simulink model "TV_2018_HIL"  (R2016a)
settings: Solver=FixedStepAuto  StartTime=0.0  StopTime=inf  FixedStep=0.001  RelTol=1e-3
PreLoadFcn:
  | TV_2017_parameters
values from neighbouring files (symbols this model uses):
  battery_voltage = single(530)    [HIL_parameters.m]    (also in HIL_parameters_2018.m; TV_2017_parameters.m; TV_2017_parameters_VD.m)
  car_params = Simulink_Car_params    [HIL_parameters.m]    (also in HIL_parameters_2018.m; TV_2017_parameters.m; TV_2017_parameters_VD.m)
  i_Diff = 16    [HIL_parameters.m]    (also in HIL_parameters_2018.m; TV_2017_parameters.m)
  Kp = 1    [HIL_parameters.m]    (also in HIL_parameters_2018.m; TV_2017_parameters.m; TV_2017_parameters_VD.m)
  motor_data = struct    [HIL_parameters.m]    (also in HIL_parameters_2018.m; TV_2017_parameters.m)
  powerLimitControl = Simulink_el    [HIL_parameters.m]    (also in HIL_parameters_2018.m; TV_2017_parameters.m; TV_2017_parameters_VD.m)
  settings = Simulink_Settings    [HIL_parameters.m]    (also in HIL_parameters_2018.m; TV_2017_parameters.m; TV_2017_parameters_VD.m)
  SpdC_BCC = 0    [HIL_parameters.m]    (also in HIL_parameters_2018.m; TV_2017_parameters.m; TV_2017_parameters_VD.m)
  Speed_Neg_sat = -21    [HIL_parameters.m]    (also in HIL_parameters_2018.m; TV_2017_parameters.m; TV_2017_parameters_VD.m)
  Speed_Pos_sat = 21    [HIL_parameters.m]    (also in HIL_parameters_2018.m; TV_2017_parameters.m; TV_2017_parameters_VD.m)
  SteeringAngleFL = [-23.80 -22.65 -21.50 -20.34 -19.18 -18.03 -16.86 -15.70 -14.53 -13.35 -12.18 -10.99 -9.80 -8.61 -7.40 -6.19 -4.97 -3.75 -2.51 -1.26 0 1.27 2.56 3.85 5.17 6.50 7.84 9.21 10.59 12.00 13.42 14.88 16.36 17.87 19.41 20.99 22.61 24.26 25.97 27.73 29.54]    [CarSetupAnalysis2018.m]    (also in HIL_parameters_2018.m; TV_2017_parameters.m; TV_2017_parameters_VD.m = [-24.129 -22.950 -21.772 -20.593 -19.413 -18.232 -17.050 -15)
  SteeringAngleFR = [-29.54 -27.73 -25.97 -24.26 -22.61 -20.99 -19.41 -17.87 -16.36 -14.88 -13.42 -12.00 -10.59 -9.21 -7.84 -6.50 -5.17 -3.85 -2.56 -1.27 0 1.26 2.51 3.75 4.97 6.19 7.40 8.61 9.80 10.99 12.18 13.35 14.53 15.70 16.86 18.03 19.18 20.34 21.50 22.65 23.80]    [CarSetupAnalysis2018.m]    (also in HIL_parameters_2018.m; TV_2017_parameters.m; TV_2017_parameters_VD.m = [-29.3050 -27.5340 -25.8140 -24.1410 -22.5110 -20.9180 -19.3)
  SteeringWhAngle = [-105 -99.75 -94.5 -89.25 -84 -78.75 -73.5 -68.25 -63 -57.75 -52.5 -47.25 -42 -36.75 -31.5 -26.25 -21.0 -15.75 -10.5 -5.25 0.0 5.25 10.50 15.75 21.00 26.25 31.50 36.75 42.00 47.25 52.50 57.75  63.00 68.25 73.50 78.75 84.00 89.25 94.50 99.75 105.00]    [TV_2017_parameters_VD.m]
  Tn_n = 0    [HIL_parameters.m]    (also in HIL_parameters_2018.m; TV_2017_parameters.m; TV_2017_parameters_VD.m)
  tractionControl = Simulink_tc    [HIL_parameters.m]    (also in HIL_parameters_2018.m; IterativeTractionControlTuning.m; TV_2017_parameters.m; TV_2017_parameters_VD.m)
  yawMomentGenerator = struct    [HIL_parameters.m]    (also in HIL_parameters_2018.m = Simulink_yawRate2; TV_2017_parameters.m = Simulink_yawRate2)
  yawRateControl = Simulink_yawRate    [HIL_parameters.m]    (also in HIL_parameters_2018.m; TV_2017_parameters.m; TV_2017_parameters_VD.m)
undefined symbols (not defined in the file or in its folder): canChannel, DiscIntNeverNeededParam, magnitude, speedEstimation, TC_Decr_Gas, TC_Derivative, TC_Incr_Gas, TC_On, TC_Relay_Off, TC_Relay_On
libraries: CarMaker4SL x366, simulink_extras x63, canmsglib x55, canlib x41, simulink x37, dspfdesign x2, sldrtlib x1
(part 2 of 15)

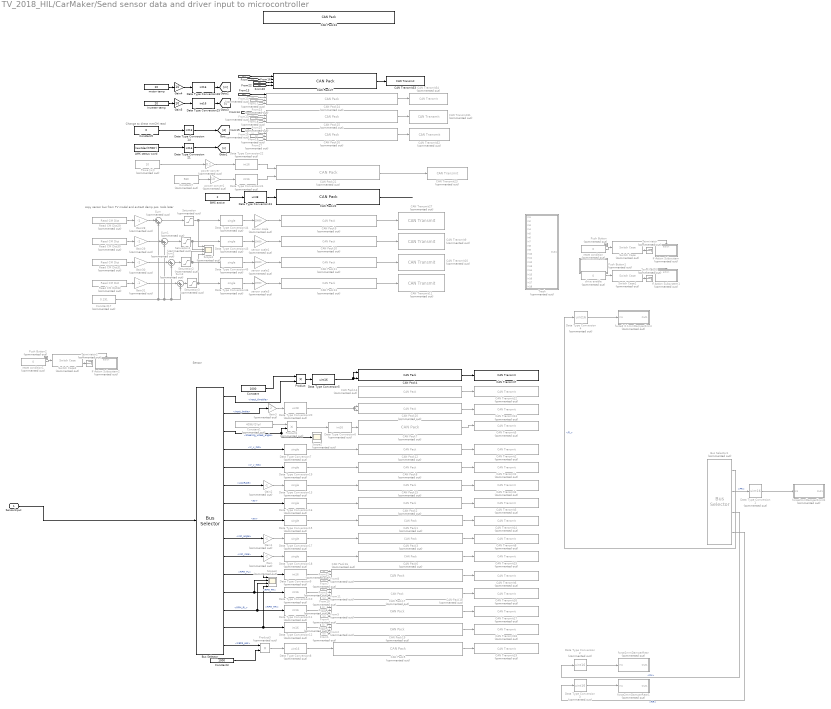
== system TV_2018_HIL/CarMaker/Send sensor data and driver input to microcontroller  ==
  note: Sensor
  note: copy sensor bus from TV model and extract damp pos. todo later
  note: Change to direct mmCM read
  SensorInput : Inport
  AMK status word : Constant  Value=hex2dec('F900')
  "BMS active " : Constant  Value=2
  Bus Selector : BusSelector  OutputSignals=Input_throttle,Input_brake,steering_wheel_angle,V_x_INS,V_y_INS,yawRate,ay,ax,roll_angle,roll_rate,RPM_FL,RPM_FR,RPM_RL,RPM_RR,KERS_pos
  Bus Selector1 : BusSelector  Commented=on  OutputSignals=FL,FR,RL,RR
  CAN Pack1 : canmsglib/CAN Pack  Commented=on  MsgList=(none)  MsgName=CAN Msg  MsgIDType=Standard (11-bit identifier)  MsgIdentifier=INS_A_X_ID  MsgLength=4  SignalInfo=Signal1$0$32$1$3$1$0$1$0$-Inf$Inf$#  NSignals=1  StartBits=str2num('[int32(0)]')  SignalSizes=str2num('[int32(32)]')  ByteOrders=str2num('[int32(1)]')  DataTypes=str2num('[int32(3)]')  MultiplexTypes=str2num('[int32(1)]')  MultiplexValues=str2num('[double(0)]')  Factors=str2num('[double(1)]')  Offsets=str2num('[double(0)]')  Minimums=str2num('[double(-Inf)]')  Maximums=str2num('[double(Inf)]')  Remote=off
      settings: DataFormat=manually specified signals
  CAN Pack10 : canmsglib/CAN Pack  Commented=on  MsgList=(none)  MsgName=ACD_DAMPER_FR_ID  MsgIDType=Standard (11-bit identifier)  MsgIdentifier=ACD_DAMPER_FR_ID  MsgLength=2  SignalInfo=Signal1$0$16$1$1$1$0$1$0$-Inf$Inf$#  NSignals=1  StartBits=str2num('[int32(0)]')  SignalSizes=str2num('[int32(16)]')  ByteOrders=str2num('[int32(1)]')  DataTypes=str2num('[int32(1)]')  MultiplexTypes=str2num('[int32(1)]')  MultiplexValues=str2num('[double(0)]')  Factors=str2num('[double(1)]')  Offsets=str2num('[double(0)]')  Minimums=str2num('[double(-Inf)]')  Maximums=str2num('[double(Inf)]')  Remote=off
      settings: DataFormat=manually specified signals
  CAN Pack11 : canmsglib/CAN Pack  Commented=on  MsgList=(none)  MsgName=ACD_DAMPER_RL_ID  MsgIDType=Standard (11-bit identifier)  MsgIdentifier=ACD_DAMPER_RL_ID  MsgLength=2  SignalInfo=Signal1$0$16$1$1$1$0$1$0$-Inf$Inf$#  NSignals=1  StartBits=str2num('[int32(0)]')  SignalSizes=str2num('[int32(16)]')  ByteOrders=str2num('[int32(1)]')  DataTypes=str2num('[int32(1)]')  MultiplexTypes=str2num('[int32(1)]')  MultiplexValues=str2num('[double(0)]')  Factors=str2num('[double(1)]')  Offsets=str2num('[double(0)]')  Minimums=str2num('[double(-Inf)]')  Maximums=str2num('[double(Inf)]')  Remote=off
      settings: DataFormat=manually specified signals
  CAN Pack12 : canmsglib/CAN Pack  Commented=on  MsgList=(none)  MsgName=CAN Msg  MsgIDType=Standard (11-bit identifier)  MsgIdentifier=INS_V_X_ID  MsgLength=4  SignalInfo=Signal1$0$32$1$3$1$0$1$0$-Inf$Inf$#  NSignals=1  StartBits=str2num('[int32(0)]')  SignalSizes=str2num('[int32(32)]')  ByteOrders=str2num('[int32(1)]')  DataTypes=str2num('[int32(3)]')  MultiplexTypes=str2num('[int32(1)]')  MultiplexValues=str2num('[double(0)]')  Factors=str2num('[double(1)]')  Offsets=str2num('[double(0)]')  Minimums=str2num('[double(-Inf)]')  Maximums=str2num('[double(Inf)]')  Remote=off
      settings: DataFormat=manually specified signals
  CAN Pack13 : canmsglib/CAN Pack  Commented=on  MsgList=(none)  MsgName=ACD_DAMPER_RR_ID  MsgIDType=Standard (11-bit identifier)  MsgIdentifier=ACD_DAMPER_RR_ID  MsgLength=2  SignalInfo=Signal1$0$16$1$1$1$0$1$0$-Inf$Inf$#  NSignals=1  StartBits=str2num('[int32(0)]')  SignalSizes=str2num('[int32(16)]')  ByteOrders=str2num('[int32(1)]')  DataTypes=str2num('[int32(1)]')  MultiplexTypes=str2num('[int32(1)]')  MultiplexValues=str2num('[double(0)]')  Factors=str2num('[double(1)]')  Offsets=str2num('[double(0)]')  Minimums=str2num('[double(-Inf)]')  Maximums=str2num('[double(Inf)]')  Remote=off
      settings: DataFormat=manually specified signals
  CAN Pack14 : canmsglib/CAN Pack  Commented=on  MsgList=(none)  MsgName=CAN Msg  MsgIDType=Standard (11-bit identifier)  MsgIdentifier=ADC_TORQUE_POSITION_RIGHT_ID  MsgLength=2  SignalInfo=APPS_R$0$16$1$2$1$0$1$0$-Inf$Inf$#  NSignals=1  StartBits=str2num('[int32(0)]')  SignalSizes=str2num('[int32(16)]')  ByteOrders=str2num('[int32(1)]')  DataTypes=str2num('[int32(2)]')  MultiplexTypes=str2num('[int32(1)]')  MultiplexValues=str2num('[double(0)]')  Factors=str2num('[double(1)]')  Offsets=str2num('[double(0)]')  Minimums=str2num('[double(-Inf)]')  Maximums=str2num('[double(Inf)]')  Remote=off
      settings: DataFormat=manually specified signals
  CAN Pack15 : canmsglib/CAN Pack  Commented=on  MsgList=(none)  MsgName=CAN Msg  MsgIDType=Standard (11-bit identifier)  MsgIdentifier=INS_YAW_RATE_ID  MsgLength=4  SignalInfo=Signal1$0$32$1$3$1$0$1$0$-Inf$Inf$#  NSignals=1  StartBits=str2num('[int32(0)]')  SignalSizes=str2num('[int32(32)]')  ByteOrders=str2num('[int32(1)]')  DataTypes=str2num('[int32(3)]')  MultiplexTypes=str2num('[int32(1)]')  MultiplexValues=str2num('[double(0)]')  Factors=str2num('[double(1)]')  Offsets=str2num('[double(0)]')  Minimums=str2num('[double(-Inf)]')  Maximums=str2num('[double(Inf)]')  Remote=off
      settings: DataFormat=manually specified signals
  CAN Pack16 : canmsglib/CAN Pack  Commented=on  MsgList=(none)  MsgName=AMK Actual Values 1  MsgIDType=Standard (11-bit identifier)  MsgIdentifier=AMK_DATA_ACTUAL_VALUE_1_FL_ID  MsgLength=8  SignalInfo=AMK_Status$0$16$1$1$1$0$1$0$-Inf$Inf$#AMK_ActualVelocity$16$16$1$1$1$0$1$0$-Inf$Inf$#AMK_TorqueCurrent$32$16$1$1$1$0$1$0$-Inf$Inf$#AMK_MagnetizingCurrent$48$16$1$1$1$0$1$0$-Inf$Inf$#  NSignals=4  StartBits=str2num('[int32(0);int32(16);int32(32);int32(48)]')  SignalSizes=str2num('[int32(16);int32(16);int32(16);int32(16)]')  ByteOrders=str2num('[int32(1);int32(1);int32(1);int32(1)]')  DataTypes=str2num('[int32(1);int32(1);int32(1);int32(1)]')  MultiplexTypes=str2num('[int32(1);int32(1);int32(1);int32(1)]')  MultiplexValues=str2num('[double(0);double(0);double(0);double(0)]')  Factors=str2num('[double(1);double(1);double(1);double(1)]')  Offsets=str2num('[double(0);double(0);double(0);double(0)]')  Minimums=str2num('[double(-Inf);double(-Inf);double(-Inf);double(-Inf)]')  Maximums=str2num('[double(Inf);double(Inf);double(Inf);double(Inf)]')  Remote=off
      settings: DataFormat=manually specified signals
  CAN Pack17 : canmsglib/CAN Pack  Commented=on  MsgList=(none)  MsgName=AMK Actual Values 1  MsgIDType=Standard (11-bit identifier)  MsgIdentifier=AMK_DATA_ACTUAL_VALUE_1_FR_ID  MsgLength=8  SignalInfo=AMK_Status$0$16$1$1$1$0$1$0$-Inf$Inf$#AMK_ActualVelocity$16$16$1$1$1$0$1$0$-Inf$Inf$#AMK_TorqueCurrent$32$16$1$1$1$0$1$0$-Inf$Inf$#AMK_MagnetizingCurrent$48$16$1$1$1$0$1$0$-Inf$Inf$#  NSignals=4  StartBits=str2num('[int32(0);int32(16);int32(32);int32(48)]')  SignalSizes=str2num('[int32(16);int32(16);int32(16);int32(16)]')  ByteOrders=str2num('[int32(1);int32(1);int32(1);int32(1)]')  DataTypes=str2num('[int32(1);int32(1);int32(1);int32(1)]')  MultiplexTypes=str2num('[int32(1);int32(1);int32(1);int32(1)]')  MultiplexValues=str2num('[double(0);double(0);double(0);double(0)]')  Factors=str2num('[double(1);double(1);double(1);double(1)]')  Offsets=str2num('[double(0);double(0);double(0);double(0)]')  Minimums=str2num('[double(-Inf);double(-Inf);double(-Inf);double(-Inf)]')  Maximums=str2num('[double(Inf);double(Inf);double(Inf);double(Inf)]')  Remote=off
      settings: DataFormat=manually specified signals
  CAN Pack18 : canmsglib/CAN Pack  Commented=on  MsgList=(none)  MsgName=AMK Actual Values 1  MsgIDType=Standard (11-bit identifier)  MsgIdentifier=AMK_DATA_ACTUAL_VALUE_1_RL_ID  MsgLength=8  SignalInfo=AMK_Status$0$16$1$1$1$0$1$0$-Inf$Inf$#AMK_ActualVelocity$16$16$1$1$1$0$1$0$-Inf$Inf$#AMK_TorqueCurrent$32$16$1$1$1$0$1$0$-Inf$Inf$#AMK_MagnetizingCurrent$48$16$1$1$1$0$1$0$-Inf$Inf$#  NSignals=4  StartBits=str2num('[int32(0);int32(16);int32(32);int32(48)]')  SignalSizes=str2num('[int32(16);int32(16);int32(16);int32(16)]')  ByteOrders=str2num('[int32(1);int32(1);int32(1);int32(1)]')  DataTypes=str2num('[int32(1);int32(1);int32(1);int32(1)]')  MultiplexTypes=str2num('[int32(1);int32(1);int32(1);int32(1)]')  MultiplexValues=str2num('[double(0);double(0);double(0);double(0)]')  Factors=str2num('[double(1);double(1);double(1);double(1)]')  Offsets=str2num('[double(0);double(0);double(0);double(0)]')  Minimums=str2num('[double(-Inf);double(-Inf);double(-Inf);double(-Inf)]')  Maximums=str2num('[double(Inf);double(Inf);double(Inf);double(Inf)]')  Remote=off
      settings: DataFormat=manually specified signals
  CAN Pack19 : canmsglib/CAN Pack  Commented=on  MsgList=(none)  MsgName=AMK Actual Values 1  MsgIDType=Standard (11-bit identifier)  MsgIdentifier=AMK_DATA_ACTUAL_VALUE_1_RR_ID  MsgLength=8  SignalInfo=AMK_Status$0$16$1$1$1$0$1$0$-Inf$Inf$#AMK_ActualVelocity$16$16$1$1$1$0$1$0$-Inf$Inf$#AMK_TorqueCurrent$32$16$1$1$1$0$1$0$-Inf$Inf$#AMK_MagnetizingCurrent$48$16$1$1$1$0$1$0$-Inf$Inf$#  NSignals=4  StartBits=str2num('[int32(0);int32(16);int32(32);int32(48)]')  SignalSizes=str2num('[int32(16);int32(16);int32(16);int32(16)]')  ByteOrders=str2num('[int32(1);int32(1);int32(1);int32(1)]')  DataTypes=str2num('[int32(1);int32(1);int32(1);int32(1)]')  MultiplexTypes=str2num('[int32(1);int32(1);int32(1);int32(1)]')  MultiplexValues=str2num('[double(0);double(0);double(0);double(0)]')  Factors=str2num('[double(1);double(1);double(1);double(1)]')  Offsets=str2num('[double(0);double(0);double(0);double(0)]')  Minimums=str2num('[double(-Inf);double(-Inf);double(-Inf);double(-Inf)]')  Maximums=str2num('[double(Inf);double(Inf);double(Inf);double(Inf)]')  Remote=off
      settings: DataFormat=manually specified signals
  CAN Pack2 : canmsglib/CAN Pack  Commented=on  MsgList=(none)  MsgName=CAN Msg  MsgIDType=Standard (11-bit identifier)  MsgIdentifier=INS_A_Y_ID  MsgLength=4  SignalInfo=Signal1$0$32$1$3$1$0$1$0$-Inf$Inf$#  NSignals=1  StartBits=str2num('[int32(0)]')  SignalSizes=str2num('[int32(32)]')  ByteOrders=str2num('[int32(1)]')  DataTypes=str2num('[int32(3)]')  MultiplexTypes=str2num('[int32(1)]')  MultiplexValues=str2num('[double(0)]')  Factors=str2num('[double(1)]')  Offsets=str2num('[double(0)]')  Minimums=str2num('[double(-Inf)]')  Maximums=str2num('[double(Inf)]')  Remote=off
      settings: DataFormat=manually specified signals
  CAN Pack20 : canmsglib/CAN Pack  Commented=on  MsgList=(none)  MsgName=CAN Msg  MsgIDType=Standard (11-bit identifier)  MsgIdentifier=ADC_BRAKE_POSITION_ID  MsgLength=2  SignalInfo=Signal1$0$8$1$1$1$0$1$0$-Inf$Inf$#Signal2$8$8$1$1$1$0$1$0$-Inf$Inf$#  NSignals=2  StartBits=str2num('[int32(0);int32(8)]')  SignalSizes=str2num('[int32(8);int32(8)]')  ByteOrders=str2num('[int32(1);int32(1)]')  DataTypes=str2num('[int32(1);int32(1)]')  MultiplexTypes=str2num('[int32(1);int32(1)]')  MultiplexValues=str2num('[double(0);double(0)]')  Factors=str2num('[double(1);double(1)]')  Offsets=str2num('[double(0);double(0)]')  Minimums=str2num('[double(-Inf);double(-Inf)]')  Maximums=str2num('[double(Inf);double(Inf)]')  Remote=off
      settings: DataFormat=manually specified signals
  CAN Pack21 : canmsglib/CAN Pack  Commented=on  MsgList=(none)  MsgName=CAN Msg  MsgIDType=Standard (11-bit identifier)  MsgIdentifier=BMS_TS_POWER  MsgLength=4  SignalInfo=power_value$0$16$1$2$1$0$1$0$-Inf$Inf$#DC_voltage$16$16$1$2$1$0$1$0$-Inf$Inf$#  NSignals=2  StartBits=str2num('[int32(0);int32(16)]')  SignalSizes=str2num('[int32(16);int32(16)]')  ByteOrders=str2num('[int32(1);int32(1)]')  DataTypes=str2num('[int32(2);int32(2)]')  MultiplexTypes=str2num('[int32(1);int32(1)]')  MultiplexValues=str2num('[double(0);double(0)]')  Factors=str2num('[double(1);double(1)]')  Offsets=str2num('[double(0);double(0)]')  Minimums=str2num('[double(-Inf);double(-Inf)]')  Maximums=str2num('[double(Inf);double(Inf)]')  Remote=off
      settings: DataFormat=manually specified signals
  CAN Pack22 : canmsglib/CAN Pack  MsgList=(none)  MsgName=CAN Msg  MsgIDType=Standard (11-bit identifier)  MsgIdentifier=BMS_STATE  MsgLength=1  SignalInfo=BMS_STATE$0$8$1$2$1$0$1$0$-Inf$Inf$#  NSignals=1  StartBits=str2num('[int32(0)]')  SignalSizes=str2num('[int32(8)]')  ByteOrders=str2num('[int32(1)]')  DataTypes=str2num('[int32(2)]')  MultiplexTypes=str2num('[int32(1)]')  MultiplexValues=str2num('[double(0)]')  Factors=str2num('[double(1)]')  Offsets=str2num('[double(0)]')  Minimums=str2num('[double(-Inf)]')  Maximums=str2num('[double(Inf)]')  Remote=off
      settings: DataFormat=manually specified signals
  CAN Pack23 : canmsglib/CAN Pack  MsgList=(none)  MsgName=AMK Actual Values 2  MsgIDType=Standard (11-bit identifier)  MsgIdentifier=AMK_DATA_ACTUAL_VALUE_2_FL_ID  MsgLength=8  SignalInfo=AMK__TempMotor$0$16$1$1$1$0$1$0$-Inf$Inf$#AMK_TempInverter$16$16$1$1$1$0$1$0$-Inf$Inf$#AMK_TorqueCurrent$32$16$1$1$1$0$1$0$-Inf$Inf$#AMK_MagnetizingCurrent$48$16$1$1$1$0$1$0$-Inf$Inf$#  NSignals=4  StartBits=str2num('[int32(0);int32(16);int32(32);int32(48)]')  SignalSizes=str2num('[int32(16);int32(16);int32(16);int32(16)]')  ByteOrders=str2num('[int32(1);int32(1);int32(1);int32(1)]')  DataTypes=str2num('[int32(1);int32(1);int32(1);int32(1)]')  MultiplexTypes=str2num('[int32(1);int32(1);int32(1);int32(1)]')  MultiplexValues=str2num('[double(0);double(0);double(0);double(0)]')  Factors=str2num('[double(1);double(1);double(1);double(1)]')  Offsets=str2num('[double(0);double(0);double(0);double(0)]')  Minimums=str2num('[double(-Inf);double(-Inf);double(-Inf);double(-Inf)]')  Maximums=str2num('[double(Inf);double(Inf);double(Inf);double(Inf)]')  Remote=off
      settings: DataFormat=manually specified signals
  CAN Pack24 : canmsglib/CAN Pack  Commented=on  MsgList=(none)  MsgName=AMK Actual Values 2  MsgIDType=Standard (11-bit identifier)  MsgIdentifier=AMK_DATA_ACTUAL_VALUE_2_FR_ID  MsgLength=8  SignalInfo=AMK__TempMotor$0$16$1$1$1$0$1$0$-Inf$Inf$#AMK_TempInverter$16$16$1$1$1$0$1$0$-Inf$Inf$#AMK_TorqueCurrent$32$16$1$1$1$0$1$0$-Inf$Inf$#AMK_MagnetizingCurrent$48$16$1$1$1$0$1$0$-Inf$Inf$#  NSignals=4  StartBits=str2num('[int32(0);int32(16);int32(32);int32(48)]')  SignalSizes=str2num('[int32(16);int32(16);int32(16);int32(16)]')  ByteOrders=str2num('[int32(1);int32(1);int32(1);int32(1)]')  DataTypes=str2num('[int32(1);int32(1);int32(1);int32(1)]')  MultiplexTypes=str2num('[int32(1);int32(1);int32(1);int32(1)]')  MultiplexValues=str2num('[double(0);double(0);double(0);double(0)]')  Factors=str2num('[double(1);double(1);double(1);double(1)]')  Offsets=str2num('[double(0);double(0);double(0);double(0)]')  Minimums=str2num('[double(-Inf);double(-Inf);double(-Inf);double(-Inf)]')  Maximums=str2num('[double(Inf);double(Inf);double(Inf);double(Inf)]')  Remote=off
      settings: DataFormat=manually specified signals
  CAN Pack25 : canmsglib/CAN Pack  Commented=on  MsgList=(none)  MsgName=AMK Actual Values 2  MsgIDType=Standard (11-bit identifier)  MsgIdentifier=AMK_DATA_ACTUAL_VALUE_2_RL_ID  MsgLength=8  SignalInfo=AMK__TempMotor$0$16$1$1$1$0$1$0$-Inf$Inf$#AMK_TempInverter$16$16$1$1$1$0$1$0$-Inf$Inf$#AMK_TorqueCurrent$32$16$1$1$1$0$1$0$-Inf$Inf$#AMK_MagnetizingCurrent$48$16$1$1$1$0$1$0$-Inf$Inf$#  NSignals=4  StartBits=str2num('[int32(0);int32(16);int32(32);int32(48)]')  SignalSizes=str2num('[int32(16);int32(16);int32(16);int32(16)]')  ByteOrders=str2num('[int32(1);int32(1);int32(1);int32(1)]')  DataTypes=str2num('[int32(1);int32(1);int32(1);int32(1)]')  MultiplexTypes=str2num('[int32(1);int32(1);int32(1);int32(1)]')  MultiplexValues=str2num('[double(0);double(0);double(0);double(0)]')  Factors=str2num('[double(1);double(1);double(1);double(1)]')  Offsets=str2num('[double(0);double(0);double(0);double(0)]')  Minimums=str2num('[double(-Inf);double(-Inf);double(-Inf);double(-Inf)]')  Maximums=str2num('[double(Inf);double(Inf);double(Inf);double(Inf)]')  Remote=off
      settings: DataFormat=manually specified signals
  CAN Pack26 : canmsglib/CAN Pack  Commented=on  MsgList=(none)  MsgName=AMK Actual Values 2  MsgIDType=Standard (11-bit identifier)  MsgIdentifier=AMK_DATA_ACTUAL_VALUE_2_RR_ID  MsgLength=8  SignalInfo=AMK__TempMotor$0$16$1$1$1$0$1$0$-Inf$Inf$#AMK_TempInverter$16$16$1$1$1$0$1$0$-Inf$Inf$#AMK_TorqueCurrent$32$16$1$1$1$0$1$0$-Inf$Inf$#AMK_MagnetizingCurrent$48$16$1$1$1$0$1$0$-Inf$Inf$#  NSignals=4  StartBits=str2num('[int32(0);int32(16);int32(32);int32(48)]')  SignalSizes=str2num('[int32(16);int32(16);int32(16);int32(16)]')  ByteOrders=str2num('[int32(1);int32(1);int32(1);int32(1)]')  DataTypes=str2num('[int32(1);int32(1);int32(1);int32(1)]')  MultiplexTypes=str2num('[int32(1);int32(1);int32(1);int32(1)]')  MultiplexValues=str2num('[double(0);double(0);double(0);double(0)]')  Factors=str2num('[double(1);double(1);double(1);double(1)]')  Offsets=str2num('[double(0);double(0);double(0);double(0)]')  Minimums=str2num('[double(-Inf);double(-Inf);double(-Inf);double(-Inf)]')  Maximums=str2num('[double(Inf);double(Inf);double(Inf);double(Inf)]')  Remote=off
      settings: DataFormat=manually specified signals
  CAN Pack27 : canmsglib/CAN Pack  MsgList=(none)  MsgName=CAN Msg  MsgIDType=Standard (11-bit identifier)  MsgIdentifier=AMK_DATA_ACTUAL_VALUE_2_FL_ID  MsgLength=8  SignalInfo=Signal1$0$16$1$1$1$0$1$0$-Inf$Inf$#Signal2$16$16$1$1$1$0$1$0$-Inf$Inf$#Signal3$32$16$1$1$1$0$1$0$-Inf$Inf$#Signal4$48$16$1$1$1$0$1$0$-Inf$Inf$#  NSignals=4  StartBits=str2num('[int32(0);int32(16);int32(32);int32(48)]')  SignalSizes=str2num('[int32(16);int32(16);int32(16);int32(16)]')  ByteOrders=str2num('[int32(1);int32(1);int32(1);int32(1)]')  DataTypes=str2num('[int32(1);int32(1);int32(1);int32(1)]')  MultiplexTypes=str2num('[int32(1);int32(1);int32(1);int32(1)]')  MultiplexValues=str2num('[double(0);double(0);double(0);double(0)]')  Factors=str2num('[double(1);double(1);double(1);double(1)]')  Offsets=str2num('[double(0);double(0);double(0);double(0)]')  Minimums=str2num('[double(-Inf);double(-Inf);double(-Inf);double(-Inf)]')  Maximums=str2num('[double(Inf);double(Inf);double(Inf);double(Inf)]')  Remote=off
      settings: DataFormat=manually specified signals
  CAN Pack3 : canmsglib/CAN Pack  Commented=on  MsgList=(none)  MsgName=CAN Msg  MsgIDType=Standard (11-bit identifier)  MsgIdentifier=INS_ROLL_ID  MsgLength=4  SignalInfo=Signal1$0$32$1$3$1$0$1$0$-Inf$Inf$#  NSignals=1  StartBits=str2num('[int32(0)]')  SignalSizes=str2num('[int32(32)]')  ByteOrders=str2num('[int32(1)]')  DataTypes=str2num('[int32(3)]')  MultiplexTypes=str2num('[int32(1)]')  MultiplexValues=str2num('[double(0)]')  Factors=str2num('[double(1)]')  Offsets=str2num('[double(0)]')  Minimums=str2num('[double(-Inf)]')  Maximums=str2num('[double(Inf)]')  Remote=off
      settings: DataFormat=manually specified signals
  CAN Pack4 : canmsglib/CAN Pack  MsgList=(none)  MsgName=CAN Msg  MsgIDType=Standard (11-bit identifier)  MsgIdentifier=ADC_TORQUE_POSITION_LEFT_ID  MsgLength=4  SignalInfo=APPS_L$0$16$1$2$1$0$1$0$-Inf$Inf$#APPS_R$16$16$1$2$1$0$1$0$-Inf$Inf$#  NSignals=2  StartBits=str2num('[int32(0);int32(16)]')  SignalSizes=str2num('[int32(16);int32(16)]')  ByteOrders=str2num('[int32(1);int32(1)]')  DataTypes=str2num('[int32(2);int32(2)]')  MultiplexTypes=str2num('[int32(1);int32(1)]')  MultiplexValues=str2num('[double(0);double(0)]')  Factors=str2num('[double(1);double(1)]')  Offsets=str2num('[double(0);double(0)]')  Minimums=str2num('[double(-Inf);double(-Inf)]')  Maximums=str2num('[double(Inf);double(Inf)]')  Remote=off
      settings: DataFormat=manually specified signals
  CAN Pack5 : canmsglib/CAN Pack  Commented=on  MsgList=(none)  MsgName=CAN Msg  MsgIDType=Standard (11-bit identifier)  MsgIdentifier=ADC_KERS_POSITION_ID  MsgLength=2  SignalInfo=KERS$0$16$1$1$1$0$1$0$-Inf$Inf$#  NSignals=1  StartBits=str2num('[int32(0)]')  SignalSizes=str2num('[int32(16)]')  ByteOrders=str2num('[int32(1)]')  DataTypes=str2num('[int32(1)]')  MultiplexTypes=str2num('[int32(1)]')  MultiplexValues=str2num('[double(0)]')  Factors=str2num('[double(1)]')  Offsets=str2num('[double(0)]')  Minimums=str2num('[double(-Inf)]')  Maximums=str2num('[double(Inf)]')  Remote=off
      settings: DataFormat=manually specified signals
  CAN Pack6 : canmsglib/CAN Pack  Commented=on  MsgList=(none)  MsgName=CAN Msg  MsgIDType=Standard (11-bit identifier)  MsgIdentifier=INS_ROLL_RATE_ID  MsgLength=4  SignalInfo=Signal1$0$32$1$3$1$0$1$0$-Inf$Inf$#  NSignals=1  StartBits=str2num('[int32(0)]')  SignalSizes=str2num('[int32(32)]')  ByteOrders=str2num('[int32(1)]')  DataTypes=str2num('[int32(3)]')  MultiplexTypes=str2num('[int32(1)]')  MultiplexValues=str2num('[double(0)]')  Factors=str2num('[double(1)]')  Offsets=str2num('[double(0)]')  Minimums=str2num('[double(-Inf)]')  Maximums=str2num('[double(Inf)]')  Remote=off
      settings: DataFormat=manually specified signals
  CAN Pack7 : canmsglib/CAN Pack  Commented=on  MsgList=(none)  MsgName=CAN Msg  MsgIDType=Standard (11-bit identifier)  MsgIdentifier=ADC_STEERING_ID  MsgLength=2  SignalInfo=steer$0$16$1$1$1$0$1$0$-Inf$Inf$#  NSignals=1  StartBits=str2num('[int32(0)]')  SignalSizes=str2num('[int32(16)]')  ByteOrders=str2num('[int32(1)]')  DataTypes=str2num('[int32(1)]')  MultiplexTypes=str2num('[int32(1)]')  MultiplexValues=str2num('[double(0)]')  Factors=str2num('[double(1)]')  Offsets=str2num('[double(0)]')  Minimums=str2num('[double(-Inf)]')  Maximums=str2num('[double(Inf)]')  Remote=off
      settings: DataFormat=manually specified signals
  CAN Pack8 : canmsglib/CAN Pack  Commented=on  MsgList=(none)  MsgName=CAN Msg  MsgIDType=Standard (11-bit identifier)  MsgIdentifier=INS_V_Y_ID  MsgLength=4  SignalInfo=Signal1$0$32$1$3$1$0$1$0$-Inf$Inf$#  NSignals=1  StartBits=str2num('[int32(0)]')  SignalSizes=str2num('[int32(32)]')  ByteOrders=str2num('[int32(1)]')  DataTypes=str2num('[int32(3)]')  MultiplexTypes=str2num('[int32(1)]')  MultiplexValues=str2num('[double(0)]')  Factors=str2num('[double(1)]')  Offsets=str2num('[double(0)]')  Minimums=str2num('[double(-Inf)]')  Maximums=str2num('[double(Inf)]')  Remote=off
      settings: DataFormat=manually specified signals
  CAN Pack9 : canmsglib/CAN Pack  Commented=on  MsgList=(none)  MsgName=CAN Msg ACD_DAMPER_FL_ID  MsgIDType=Standard (11-bit identifier)  MsgIdentifier=ACD_DAMPER_FL_ID  MsgLength=2  SignalInfo=Signal1$0$16$1$1$1$0$1$0$-Inf$Inf$#  NSignals=1  StartBits=str2num('[int32(0)]')  SignalSizes=str2num('[int32(16)]')  ByteOrders=str2num('[int32(1)]')  DataTypes=str2num('[int32(1)]')  MultiplexTypes=str2num('[int32(1)]')  MultiplexValues=str2num('[double(0)]')  Factors=str2num('[double(1)]')  Offsets=str2num('[double(0)]')  Minimums=str2num('[double(-Inf)]')  Maximums=str2num('[double(Inf)]')  Remote=off
      settings: DataFormat=manually specified signals
  CAN Transmit1 : canlib/CAN Transmit  Commented=on  BlockHandle=19056.0004  DeviceMenu=Kvaser Virtual 1 (Channel 1)  Device=PEAK-System PCAN-USB (PCAN_USBBUS1)  ObjConstructor=canChannel('PEAK-System', 'PCAN_PCIBUS1')  EnablePeriodicTransmit=off  MessagePeriod=1.000
  CAN Transmit10 : canlib/CAN Transmit  Commented=on  BlockHandle=19057.0006  DeviceMenu=Kvaser Virtual 1 (Channel 1)  Device=PEAK-System PCAN-USB (PCAN_USBBUS1)  ObjConstructor=canChannel('PEAK-System', 'PCAN_PCIBUS1')  EnablePeriodicTransmit=off  MessagePeriod=1.000
  CAN Transmit11 : canlib/CAN Transmit  Commented=on  BlockHandle=19058.0011  DeviceMenu=Kvaser Virtual 1 (Channel 1)  Device=PEAK-System PCAN-USB (PCAN_USBBUS1)  ObjConstructor=canChannel('PEAK-System', 'PCAN_PCIBUS1')  EnablePeriodicTransmit=off  MessagePeriod=1.000
  CAN Transmit12 : canlib/CAN Transmit  Commented=on  BlockHandle=19059.0004  DeviceMenu=Kvaser Virtual 1 (Channel 1)  Device=PEAK-System PCAN-USB (PCAN_USBBUS1)  ObjConstructor=canChannel('PEAK-System', 'PCAN_PCIBUS1')  EnablePeriodicTransmit=off  MessagePeriod=1.000
  CAN Transmit13 : canlib/CAN Transmit  Commented=on  BlockHandle=19060.0004  DeviceMenu=Kvaser Virtual 1 (Channel 1)  Device=PEAK-System PCAN-USB (PCAN_USBBUS1)  ObjConstructor=canChannel('PEAK-System', 'PCAN_PCIBUS1')  EnablePeriodicTransmit=off  MessagePeriod=1.000
  CAN Transmit14 : canlib/CAN Transmit  Commented=on  BlockHandle=19061.0004  DeviceMenu=Kvaser Virtual 1 (Channel 1)  Device=PEAK-System PCAN-USB (PCAN_USBBUS1)  ObjConstructor=canChannel('PEAK-System', 'PCAN_PCIBUS1')  EnablePeriodicTransmit=off  MessagePeriod=1.000
  CAN Transmit15 : canlib/CAN Transmit  Commented=on  BlockHandle=19062.0006  DeviceMenu=Kvaser Virtual 1 (Channel 1)  Device=PEAK-System PCAN-USB (PCAN_USBBUS1)  ObjConstructor=canChannel('PEAK-System', 'PCAN_PCIBUS1')  EnablePeriodicTransmit=off  MessagePeriod=1.000
  CAN Transmit16 : canlib/CAN Transmit  Commented=on  BlockHandle=19063.0011  DeviceMenu=Kvaser Virtual 1 (Channel 1)  Device=PEAK-System PCAN-USB (PCAN_USBBUS1)  ObjConstructor=canChannel('PEAK-System', 'PCAN_PCIBUS1')  EnablePeriodicTransmit=off  MessagePeriod=1.000
  CAN Transmit17 : canlib/CAN Transmit  Commented=on  BlockHandle=19064.0004  DeviceMenu=Kvaser Virtual 1 (Channel 1)  Device=PEAK-System PCAN-USB (PCAN_USBBUS1)  ObjConstructor=canChannel('PEAK-System', 'PCAN_PCIBUS1')  EnablePeriodicTransmit=off  MessagePeriod=1.000
  CAN Transmit18 : canlib/CAN Transmit  Commented=on  BlockHandle=19065.0004  DeviceMenu=Kvaser Virtual 1 (Channel 1)  Device=PEAK-System PCAN-USB (PCAN_USBBUS1)  ObjConstructor=canChannel('PEAK-System', 'PCAN_PCIBUS1')  EnablePeriodicTransmit=off  MessagePeriod=1.000
  CAN Transmit19 : canlib/CAN Transmit  Commented=on  BlockHandle=19066.0004  DeviceMenu=Kvaser Virtual 1 (Channel 1)  Device=PEAK-System PCAN-USB (PCAN_USBBUS1)  ObjConstructor=canChannel('PEAK-System', 'PCAN_PCIBUS1')  EnablePeriodicTransmit=off  MessagePeriod=1.000
  CAN Transmit2 : canlib/CAN Transmit  Commented=on  BlockHandle=19067.0006  DeviceMenu=Kvaser Virtual 1 (Channel 1)  Device=PEAK-System PCAN-USB (PCAN_USBBUS1)  ObjConstructor=canChannel('PEAK-System', 'PCAN_PCIBUS1')  EnablePeriodicTransmit=off  MessagePeriod=1.000
  CAN Transmit23 : canlib/CAN Transmit  Commented=on  BlockHandle=19068.0011  DeviceMenu=Kvaser Virtual 1 (Channel 1)  Device=PEAK-System PCAN-USB (PCAN_USBBUS1)  ObjConstructor=canChannel('PEAK-System', 'PCAN_PCIBUS1')  EnablePeriodicTransmit=off  MessagePeriod=1.000
  CAN Transmit27 : canlib/CAN Transmit  Commented=on  BlockHandle=19069.0004  DeviceMenu=Kvaser Virtual 1 (Channel 1)  Device=PEAK-System PCAN-USB (PCAN_USBBUS1)  ObjConstructor=canChannel('PEAK-System', 'PCAN_PCIBUS1')  EnablePeriodicTransmit=off  MessagePeriod=1.000
  CAN Transmit3 : canlib/CAN Transmit  Commented=on  BlockHandle=19070.0004  DeviceMenu=Kvaser Virtual 1 (Channel 1)  Device=PEAK-System PCAN-USB (PCAN_USBBUS1)  ObjConstructor=canChannel('PEAK-System', 'PCAN_PCIBUS1')  EnablePeriodicTransmit=off  MessagePeriod=1.000
  CAN Transmit31 : canlib/CAN Transmit  Commented=on  BlockHandle=19071.0004  DeviceMenu=Kvaser Virtual 1 (Channel 1)  Device=PEAK-System PCAN-USB (PCAN_USBBUS1)  ObjConstructor=canChannel('PEAK-System', 'PCAN_PCIBUS1')  EnablePeriodicTransmit=off  MessagePeriod=1.000
  CAN Transmit32 : canlib/CAN Transmit  Commented=on  BlockHandle=19072.0006  DeviceMenu=Kvaser Virtual 1 (Channel 1)  Device=PEAK-System PCAN-USB (PCAN_USBBUS1)  ObjConstructor=canChannel('PEAK-System', 'PCAN_PCIBUS1')  EnablePeriodicTransmit=off  MessagePeriod=1.000
  CAN Transmit33 : canlib/CAN Transmit  BlockHandle=19073.0011  DeviceMenu=Kvaser Virtual 1 (Channel 1)  Device=PEAK-System PCAN-USB (PCAN_USBBUS1)  ObjConstructor=canChannel('PEAK-System', 'PCAN_PCIBUS1')  EnablePeriodicTransmit=off  MessagePeriod=1.000
  CAN Transmit34 : canlib/CAN Transmit  Commented=on  BlockHandle=19074.0004  DeviceMenu=Kvaser Virtual 1 (Channel 1)  Device=PEAK-System PCAN-USB (PCAN_USBBUS1)  ObjConstructor=canChannel('PEAK-System', 'PCAN_PCIBUS1')  EnablePeriodicTransmit=off  MessagePeriod=1.000
  CAN Transmit4 : canlib/CAN Transmit  Commented=on  BlockHandle=19075.0004  DeviceMenu=Kvaser Virtual 1 (Channel 1)  Device=PEAK-System PCAN-USB (PCAN_USBBUS1)  ObjConstructor=canChannel('PEAK-System', 'PCAN_PCIBUS1')  EnablePeriodicTransmit=off  MessagePeriod=1.000
  CAN Transmit5 : canlib/CAN Transmit  Commented=on  BlockHandle=19076.0004  DeviceMenu=Kvaser Virtual 1 (Channel 1)  Device=PEAK-System PCAN-USB (PCAN_USBBUS1)  ObjConstructor=canChannel('PEAK-System', 'PCAN_PCIBUS1')  EnablePeriodicTransmit=off  MessagePeriod=1.000
  CAN Transmit6 : canlib/CAN Transmit  Commented=on  BlockHandle=19077.0006  DeviceMenu=Kvaser Virtual 1 (Channel 1)  Device=PEAK-System PCAN-USB (PCAN_USBBUS1)  ObjConstructor=canChannel('PEAK-System', 'PCAN_PCIBUS1')  EnablePeriodicTransmit=off  MessagePeriod=1.000
  CAN Transmit7 : canlib/CAN Transmit  BlockHandle=19078.0011  DeviceMenu=Kvaser Virtual 1 (Channel 1)  Device=PEAK-System PCAN-USB (PCAN_USBBUS1)  ObjConstructor=canChannel('PEAK-System', 'PCAN_PCIBUS1')  EnablePeriodicTransmit=off  MessagePeriod=1.000
  CAN Transmit8 : canlib/CAN Transmit  Commented=on  BlockHandle=19079.0004  DeviceMenu=Kvaser Virtual 1 (Channel 1)  Device=PEAK-System PCAN-USB (PCAN_USBBUS1)  ObjConstructor=canChannel('PEAK-System', 'PCAN_PCIBUS1')  EnablePeriodicTransmit=off  MessagePeriod=1.000
  CAN Transmit9 : canlib/CAN Transmit  Commented=on  BlockHandle=19080.0004  DeviceMenu=Kvaser Virtual 1 (Channel 1)  Device=PEAK-System PCAN-USB (PCAN_USBBUS1)  ObjConstructor=canChannel('PEAK-System', 'PCAN_PCIBUS1')  EnablePeriodicTransmit=off  MessagePeriod=1.000
  Constant : Constant  Value=1000
  Constant1 : Constant  Commented=on  Value=4096/(2*pi)
  Constant17 : Constant  Commented=on  Value=0.191
  Constant3 : Constant  Value=1000  OutDataTypeStr=single
  Constant5 : Constant  Value=0
  Constant7 : Constant  Commented=on  Value=580
  Data Type Conversion1 : DataTypeConversion  Commented=on  OutDataTypeStr=uint16
  Data Type Conversion{6,9..12,22,24} (7 alike) : DataTypeConversion  Commented=on  OutDataTypeStr=int16
  Data Type Conversion{7,13,15..19,43..46} (11 alike) : DataTypeConversion  Commented=on  OutDataTypeStr=single
  Data Type Conversion{14,21,25,28} (4 alike) : DataTypeConversion  OutDataTypeStr=int16
  Data Type Conversion2 : DataTypeConversion  Commented=on  OutDataTypeStr=uint16
  Data Type Conversion20 : DataTypeConversion  Commented=on  OutDataTypeStr=uint8
  Data Type Conversion23 : DataTypeConversion  OutDataTypeStr=uint8
  Data Type Conversion3 : DataTypeConversion  Commented=on  OutDataTypeStr=uint16  SaturateOnIntegerOverflow=on
  Data Type Conversion4 : DataTypeConversion  Commented=on  OutDataTypeStr=uint16
  Data Type Conversion5 : DataTypeConversion  OutDataTypeStr=uint16
  Data Type Conversion8 : DataTypeConversion  Commented=on  OutDataTypeStr=uint16  SaturateOnIntegerOverflow=on
  From{1..2,4..5,7..8,10..11,21,23..27} (14 alike) : From  Commented=on
  From{3,6,9,12} (4 alike) : From  Commented=on  GotoTag=s
  From17 : From  Commented=on  GotoTag=i
  From18 : From  Commented=on  GotoTag=i
  From19 : From  Commented=on  GotoTag=i
  Gain{,1..2,28..31} (7 alike) : Gain  Commented=on  Gain=-1
  Gain3 : Gain  Commented=on  Gain=2
  Gain4 : Gain  Gain=10
  Gain5 : Gain  Gain=10
  If Action Subsystem : Subsystem  Commented=on  TreatAsAtomicUnit=on
  If Action Subsystem1 : Subsystem  Commented=on  TreatAsAtomicUnit=on
  If Action Subsystem2 : Subsystem  Commented=on  TreatAsAtomicUnit=on
  Inverter temp : Constant  Value=20  OutDataTypeStr=single
  "Powe [w]r " : Constant  Commented=on  Value=10
  Product : Product
  Product1 : Product  Commented=on
  Product3 : Product  Commented=on  OutDataTypeStr=double
  Push Button : Subsystem  Commented=on  DialogController=hmiCreateDDGDialog  IsWebBlock=on  mask(MWDashboardBlock){webBlockId=700a7f0b-a3b4-4dcb-9764-000880f57d4f, webBlockType=pushbutton, ShowInLibBrwoser=on, ShowInitialText=on, HMISrcModelName=TV_2018_HIL}
      mask prompts: webBlockId "WebBlock Id"; webBlockType "WebBlock Type"; HMISrcModelName "Source Model"
      mask Help: helpview([docroot '/mapfiles/simulink.map'], 'hmi_push_button')
      mask Display:
      | model = bdroot(gcb);
      | if strcmp(get_param(model,'BlockDiagramType'), 'library')
      |     image([(matlabroot) '/toolbox/simulink/hmi/icons/PushButton.png']);
      | end
  Push Button1 : Subsystem  Commented=on  DialogController=hmiCreateDDGDialog  IsWebBlock=on  mask(MWDashboardBlock){webBlockId=b6dae986-094a-487b-a7f2-31e17e42e774, webBlockType=pushbutton, ShowInLibBrwoser=on, ShowInitialText=on, HMISrcModelName=TV_2018_HIL}
      mask prompts: webBlockId "WebBlock Id"; webBlockType "WebBlock Type"; HMISrcModelName "Source Model"
      mask Help: helpview([docroot '/mapfiles/simulink.map'], 'hmi_push_button')
      mask Display:
      | model = bdroot(gcb);
      | if strcmp(get_param(model,'BlockDiagramType'), 'library')
      |     image([(matlabroot) '/toolbox/simulink/hmi/icons/PushButton.png']);
      | end
  Push Button2 : Subsystem  Commented=on  DialogController=hmiCreateDDGDialog  IsWebBlock=on  mask(MWDashboardBlock){webBlockId=70fa724c-954a-4912-ae00-33dd4a566d27, webBlockType=pushbutton, ShowInLibBrwoser=on, ShowInitialText=on, HMISrcModelName=TV_2018_HIL}
      mask prompts: webBlockId "WebBlock Id"; webBlockType "WebBlock Type"; HMISrcModelName "Source Model"
      mask Help: helpview([docroot '/mapfiles/simulink.map'], 'hmi_push_button')
      mask Display:
      | model = bdroot(gcb);
      | if strcmp(get_param(model,'BlockDiagramType'), 'library')
      |     image([(matlabroot) '/toolbox/simulink/hmi/icons/PushButton.png']);
      | end
  Read CM Dict29 : CarMaker4SL/Read CM Dict  Commented=on  xname=Car.SpringFL.l  xsync=off
  Read CM Dict30 : CarMaker4SL/Read CM Dict  Commented=on  xname=Car.SpringFR.l  xsync=off
  Read CM Dict31 : CarMaker4SL/Read CM Dict  Commented=on  xname=Car.SpringRL.l  xsync=off
  Read CM Dict32 : CarMaker4SL/Read CM Dict  Commented=on  xname=Car.SpringRR.l  xsync=off
  Saturation{,1..3} (4 alike) : Saturate  Commented=on  UpperLimit=0.2  LowerLimit=0.001
  Scope1 : Scope  Commented=on  NumInputPorts=4
  Scope2 : Scope  Commented=on
  Scope3 : Scope  Commented=on  NumInputPorts=4
  Sum{,1..3} (4 alike) : Sum  Commented=on  Inputs=|++
  Switch Case : SwitchCase  Commented=on
  Switch Case1 : SwitchCase  Commented=on
  Switch Case2 : SwitchCase  Commented=on
  Terminator : Terminator  Commented=on
  Terminator1 : Terminator  Commented=on
  Terminator2 : Terminator  Commented=on
  Trash : Subsystem  Commented=on
  drive enable : Constant  Commented=on  Value=0
  force2 0.1mmDamperFront : Subsystem  Commented=on
  force2mmDamperFront1 : Subsystem  Commented=on
  force2mmDamperRear : Subsystem  Commented=on
  force2mmDamperRear1 : Subsystem  Commented=on
  motor temp : Constant  Value=20  OutDataTypeStr=single
  power conver : Gain  Commented=on  Gain=0.1
  power conver1 : Gain  Commented=on  Gain=10
  reset condition : Constant  Commented=on  Value=0
  reset condition1 : Constant  Commented=on  Value=0
  sensor scale{,1..3} (4 alike) : Gain  Commented=on  Gain=10000
  wires:
  sensor scale/1 -> CAN Pack9/1
  Switch Case/1 -> If Action Subsystem/Action
  Switch Case/2 -> Terminator/1
  reset condition/1 -> Switch Case/1
  Switch Case1/1 -> If Action Subsystem1/Action
  Switch Case1/2 -> Terminator1/1
  drive enable/1 -> Switch Case1/1
  Read CM Dict30/1 -> Gain29/1
  Read CM Dict31/1 -> Gain30/1
  Read CM Dict32/1 -> Gain31/1
  Read CM Dict29/1 -> Gain28/1
  Sum/1 -> Saturation/1
  Gain28/1 -> Sum/1
  Gain29/1 -> Sum1/1
  Gain30/1 -> Sum2/1
  Gain31/1 -> Sum3/1
  Constant17/1 -> Sum3/2, Sum2/2, Sum1/2, Sum/2
  Sum1/1 -> Saturation1/1
  Sum2/1 -> Saturation2/1
  Sum3/1 -> Saturation3/1
  Saturation/1 -> Scope1/1, Data Type Conversion44/1
  Saturation1/1 -> Scope1/2, Data Type Conversion43/1
  Saturation2/1 -> Scope1/3, Data Type Conversion45/1
  Saturation3/1 -> Scope1/4, Data Type Conversion46/1
  Bus Selector1/1 -> Data Type Conversion4/1  "<FL>"
  Bus Selector1/2 -> Data Type Conversion1/1  "<FR>"
  Bus Selector1/4 -> Data Type Conversion3/1  "<RR>"
  Bus Selector1/3 -> Data Type Conversion2/1  "<RL>"
  Data Type Conversion4/1 -> force2 0.1mmDamperFront/1(In1)
  Data Type Conversion1/1 -> force2mmDamperFront1/1(In1)
  Data Type Conversion2/1 -> force2mmDamperRear/1(In1)
  Data Type Conversion3/1 -> force2mmDamperRear1/1(In1)
  sensor scale1/1 -> CAN Pack10/1
  sensor scale2/1 -> CAN Pack11/1
  sensor scale3/1 -> CAN Pack13/1
  Data Type Conversion44/1 -> sensor scale/1
  Data Type Conversion43/1 -> sensor scale1/1
  Data Type Conversion45/1 -> sensor scale2/1
  Data Type Conversion46/1 -> sensor scale3/1
  ? -> ?
  ? -> ?
  Data Type Conversion12/1 -> CAN Pack19/2
  CAN Pack8/1 -> CAN Transmit1/1
  Data Type Conversion7/1 -> CAN Pack12/1
  Gain2/1 -> Data Type Conversion13/1
  Data Type Conversion8/1 -> CAN Pack5/1
  Product3/1 -> Data Type Conversion8/1
  CAN Pack12/1 -> CAN Transmit2/1
  CAN Pack6/1 -> CAN Transmit15/1
  Data Type Conversion17/1 -> CAN Pack3/1
  Gain1/1 -> Data Type Conversion17/1
  Data Type Conversion18/1 -> CAN Pack6/1
  CAN Pack3/1 -> CAN Transmit8/1
  Data Type Conversion20/1 -> CAN Pack20/2, CAN Pack20/1
  Gain/1 -> Data Type Conversion18/1
  Bus Selector/4 -> Data Type Conversion7/1  "<V_x_INS>"
  Data Type Conversion19/1 -> CAN Pack8/1
  Gain3/1 -> Data Type Conversion20/1
  CAN Pack20/1 -> CAN Transmit13/1
  Bus Selector/6 -> Gain2/1  "<yawRate>"
  Data Type Conversion16/1 -> CAN Pack2/1
  CAN Pack1/1 -> CAN Transmit14/1
  Data Type Conversion11/1 -> CAN Pack18/2
  CAN Pack16/1 -> CAN Transmit6/1
  From10/1 -> CAN Pack17/3
  From12/1 -> CAN Pack16/1
  From5/1 -> CAN Pack18/4
  CAN Pack18/1 -> CAN Transmit17/1
  From4/1 -> CAN Pack18/3
  From1/1 -> CAN Pack19/3
  Data Type Conversion13/1 -> CAN Pack15/1
  From7/1 -> CAN Pack16/3
  From11/1 -> CAN Pack17/4
  From9/1 -> CAN Pack19/1
  From2/1 -> CAN Pack19/4
  From8/1 -> CAN Pack16/4
  CAN Pack15/1 -> CAN Transmit4/1
  CAN Pack19/1 -> CAN Transmit18/1
  Data Type Conversion9/1 -> CAN Pack16/2
  CAN Pack14/1 -> CAN Transmit12/1
  CAN Pack17/1 -> CAN Transmit16/1
  CAN Pack2/1 -> CAN Transmit3/1
  Data Type Conversion15/1 -> CAN Pack1/1
  From6/1 -> CAN Pack18/1
  From3/1 -> CAN Pack17/1
  Data Type Conversion10/1 -> CAN Pack17/2
  Product1/1 -> Data Type Conversion6/1
  Constant1/1 -> Product1/1
  Constant/1 -> Product/1
  CAN Pack4/1 -> CAN Transmit7/1
  Constant3/1 -> Product3/2
  Data Type Conversion6/1 -> CAN Pack7/1
  Product/1 -> Data Type Conversion5/1
  CAN Pack7/1 -> CAN Transmit5/1
  CAN Pack5/1 -> CAN Transmit19/1
  Data Type Conversion5/1 -> CAN Pack4/2, CAN Pack4/1
  Bus Selector/15 -> Product3/1  "<KERS_pos>"
  Bus Selector/13 -> Scope3/3, Data Type Conversion11/1  "<RPM_RL>"
  Bus Selector/2 -> Gain3/1  "<Input_brake>"
  Bus Selector/1 -> Product/2  "<Input_throttle>"
  Bus Selector/14 -> Data Type Conversion12/1, Scope3/4  "<RPM_RR>"
  Bus Selector/12 -> Scope3/2, Data Type Conversion10/1  "<RPM_FR>"
  Bus Selector/5 -> Data Type Conversion19/1  "<V_y_INS>"
  Bus Selector/10 -> Gain/1  "<roll_rate>"
  Bus Selector/9 -> Gain1/1  "<roll_angle>"
  Bus Selector/8 -> Data Type Conversion15/1  "<ax>"
  Bus Selector/11 -> Scope3/1, Data Type Conversion9/1  "<RPM_FL>"
  Bus Selector/7 -> Data Type Conversion16/1  "<ay>"
  Bus Selector/3 -> Scope2/1, Product1/2  "<steering_wheel_angle>"
  SensorInput/1 -> Bus Selector/1
  Switch Case2/1 -> If Action Subsystem2/Action
  Switch Case2/2 -> Terminator2/1
  reset condition1/1 -> Switch Case2/1
  CAN Pack9/1 -> CAN Transmit27/1
  CAN Pack10/1 -> CAN Transmit9/1
  CAN Pack11/1 -> CAN Transmit10/1
  CAN Pack13/1 -> CAN Transmit11/1
  Constant5/1 -> Data Type Conversion14/1
  Data Type Conversion14/1 -> [A]
  AMK status word/1 -> Data Type Conversion21/1
  Data Type Conversion21/1 -> [s]
  CAN Pack21/1 -> CAN Transmit23/1
  Data Type Conversion22/1 -> CAN Pack21/1
  "Powe [w]r "/1 -> power conver/1
  CAN Pack22/1 -> ?
  Data Type Conversion23/1 -> CAN Pack22/1
  "BMS active "/1 -> Data Type Conversion23/1
  Constant7/1 -> power conver1/1
  Data Type Conversion24/1 -> CAN Pack21/2
  power conver/1 -> Data Type Conversion22/1
  power conver1/1 -> Data Type Conversion24/1
  CAN Pack27/1 -> CAN Transmit33/1
  CAN Pack24/1 -> CAN Transmit34/1
  CAN Pack25/1 -> CAN Transmit31/1
  CAN Pack26/1 -> CAN Transmit32/1
  motor temp/1 -> Gain4/1
  Gain4/1 -> Data Type Conversion28/1
  Inverter temp/1 -> Gain5/1
  Gain5/1 -> Data Type Conversion25/1
  Data Type Conversion28/1 -> [m]
  Data Type Conversion25/1 -> [i]
  [m] -> CAN Pack24/1
  [m] -> CAN Pack25/1
  [m] -> CAN Pack26/1
  From17/1 -> CAN Pack24/2
  From18/1 -> CAN Pack25/2
  From19/1 -> CAN Pack26/2
  [A] -> CAN Pack27/3
  From21/1 -> CAN Pack24/3
  [A] -> CAN Pack27/4
  From23/1 -> CAN Pack24/4
  From24/1 -> CAN Pack25/3
  From25/1 -> CAN Pack25/4
  From26/1 -> CAN Pack26/3
  From27/1 -> CAN Pack26/4
  [i] -> CAN Pack27/2
  [m] -> CAN Pack27/1

== system TV_2018_HIL/CarMaker/Subsystem ==
  In1 : Inport
  "Control Output to CarMaker model " : Subsystem  Commented=on
  "Control_System " : Subsystem  Commented=on  TreatAsAtomicUnit=on
  "Debug Information " : Subsystem  Commented=on
  Estimations : Subsystem  Commented=on  TreatAsAtomicUnit=on
  From6 : From  Commented=on  GotoTag=sensors
  Out1 : Outport
  Out2 : Outport  Port=2
  Out3 : Outport  Port=3
  Out4 : Outport  Port=4
  wires:
  "Control_System "/1("Ti_pos ") -> "Control Output to CarMaker model "/1("Ti_pos ")
  "Control_System "/2(Ti_neg) -> "Control Output to CarMaker model "/2(Ti_neg)
  "Control_System "/3(wi_sp) -> "Control Output to CarMaker model "/3(wi_ref)
  Estimations/1(States) -> "Control_System "/1("States "), "Debug Information "/2(states)
  Estimations/2(whl_v) -> "Debug Information "/3(whl_speed)
  Estimations/3(Fx) -> "Debug Information "/4(Fx_est)
  Estimations/4(SR) -> "Debug Information "/5("SR ")
  Estimations/5(normLongTireForce) -> "Debug Information "/7(norm_long_tire_force)
  From6/1 -> "Debug Information "/6(Sensors)
  "Control_System "/4(TV_monitoring) -> "Debug Information "/1(TV_monitoring)
  Estimations/9(FZ_acc) -> "Debug Information "/8(Fz_acc)
  Estimations/8(alfa_r) -> Out3/1
  Estimations/6(OutputTelemetri_est) -> Out1/1
  Estimations/10("Alfa_r_acc ") -> Out4/1
  Estimations/7(T_motor) -> Out2/1
  In1/1 -> Estimations/1(Sensors_in)
